simulink model "GS_model"  (R2018b)
settings: Solver=ode5  StartTime=0.0  StopTime=SimuStopTime  FixedStep=T_Simu  RelTol=1e-3
InitFcn:
  | Initial
undefined symbols (not defined in the file or in its folder): Aba10, Aba20, aeroCIP2006_S, aeroCIP2006_X, aeroCIP2006_Y, Agl0, Ass_kS, Ass_n1, Ass_n2, Ass_n3, Ass_n4, Ass_Noise, Ass_R, Ass_Resolution, Ass_TmOrder, AssA_Fix_Abs, AssB_Fix_Abs, AssC_Fix_Abs, AssD_Fix_Abs, AssE_Fix_Aps, AssF_Fix_Aps, C, c_max, c_min, Cd, CenterOfFigNX, CenterOfFigNY, CenterOfFigNZ, CenterOfFigP1, CenterOfFigP2, CenterOfFigPX, CenterOfFigPY, CenterOfFigPZ, Cmu, Crou, DEG2RAD, DiscIntNeverNeededParam, Eg_Dir, Eg_F, Eg_PrepareTime, Eg_r_L_L, Fw_Abf, Fw_Hmax, Fw_J, Fw_Spd0, Fw_Tmax, git_hash_BaseLine, git_hash_Project, Gnss_Noise_Pos, Gnss_Noise_Vel, Gnss_PropgationTime, GyroA_Fix_Abg, GyroA_Noise, GyroB_Fix_Abg, GyroB_Noise, GyroC_Fix_Abg, GyroC_Noise, GyroD_Fix_Abg, GyroD_Noise, h ... (+94)
libraries: simulink x308, sharedutil x46, aerolibutil x37, sharedtransform x31, vrlib x14, aerolibgravity2 x2
(part 2 of 20)

== system GS_model/Subsystem2/Tc/Fw2 ==
  FwSpd0 : Inport
  In1 : Inport  Port=2
  Constant : Constant  Value=[0;0;zeros(14,1);0]
  Constant1 : Constant  Value=TestMode
  Constant2 : Constant  Value=TestMode
  Constant3 : Constant  Value=Fw_Spd0
  Data Store Memory : DataStoreMemory  DataStoreName=Dyn_FWSpdSet  ReadBeforeWriteMsg=warning  WriteAfterWriteMsg=warning  WriteAfterReadMsg=warning  InitialValue=[0;0;0]  ShowAdditionalParam=off
  Data Store Memory1 : DataStoreMemory  DataStoreName=Dyn_FWCtrlSourceSet  ReadBeforeWriteMsg=warning  WriteAfterWriteMsg=warning  WriteAfterReadMsg=warning  InitialValue=[0;0]  ShowAdditionalParam=off
  Data Store Memory10 : DataStoreMemory  DataStoreName=Dyn_FWErr_TOP  ReadBeforeWriteMsg=warning  WriteAfterWriteMsg=warning  WriteAfterReadMsg=warning  InitialValue=[0;0]  ShowAdditionalParam=off
  Data Store Memory14 : DataStoreMemory  DataStoreName=Dyn_FwFricCoff  ReadBeforeWriteMsg=warning  WriteAfterWriteMsg=warning  WriteAfterReadMsg=warning  InitialValue=1  ShowAdditionalParam=off
  Data Store Memory17 : DataStoreMemory  DataStoreName=Dyn_FWTSet  ReadBeforeWriteMsg=warning  WriteAfterWriteMsg=warning  WriteAfterReadMsg=warning  InitialValue=[0;0;0]  ShowAdditionalParam=off
  Data Store Memory2 : DataStoreMemory  DataStoreName=Dyn_FWErr_SpdOP  ReadBeforeWriteMsg=warning  WriteAfterWriteMsg=warning  WriteAfterReadMsg=warning  InitialValue=[0;0]  ShowAdditionalParam=off
  Data Store Memory3 : DataStoreMemory  DataStoreName=FwSpd0  ReadBeforeWriteMsg=warning  WriteAfterWriteMsg=warning  WriteAfterReadMsg=warning  InitialValue=Fw_Spd0  ShowAdditionalParam=off
  Data Store Memory4 : DataStoreMemory  DataStoreName=Dyn_FwDelaySet  ReadBeforeWriteMsg=warning  WriteAfterWriteMsg=warning  WriteAfterReadMsg=warning  ShowAdditionalParam=off
  Data Store Memory6 : DataStoreMemory  DataStoreName=Dyn_FWModeSet  ReadBeforeWriteMsg=warning  WriteAfterWriteMsg=warning  WriteAfterReadMsg=warning  InitialValue=[0;0;0]  ShowAdditionalParam=off
  Data Store Read : DataStoreRead  DataStoreName=Dyn_FWSpdSet
  Data Store Read1 : DataStoreRead  DataStoreName=Dyn_FWCtrlSourceSet
  Data Store Read10 : DataStoreRead  DataStoreName=Dyn_FWErr_TOP
  Data Store Read14 : DataStoreRead  DataStoreName=Dyn_FwFricCoff
  Data Store Read17 : DataStoreRead  DataStoreName=Dyn_FWTSet
  Data Store Read2 : DataStoreRead  DataStoreName=Dyn_FWErr_SpdOP
  Data Store Read3 : DataStoreRead  DataStoreName=FwSpd0
  Data Store Read4 : DataStoreRead  DataStoreName=Dyn_FwDelaySet
  Data Store Read6 : DataStoreRead  DataStoreName=Dyn_FWModeSet
  Data Store Write : DataStoreWrite  DataStoreName=Dyn_FWSpdSet
  Data Store Write1 : DataStoreWrite  DataStoreName=Dyn_FWCtrlSourceSet
  Data Store Write10 : DataStoreWrite  DataStoreName=Dyn_FWErr_TOP
  Data Store Write14 : DataStoreWrite  DataStoreName=Dyn_FwFricCoff
  Data Store Write17 : DataStoreWrite  DataStoreName=Dyn_FWTSet
  Data Store Write2 : DataStoreWrite  DataStoreName=FwSpd0
  Data Store Write4 : DataStoreWrite  DataStoreName=Dyn_FwDelaySet
  Data Store Write6 : DataStoreWrite  DataStoreName=Dyn_FWModeSet
  Data Store Write8 : DataStoreWrite  DataStoreName=Dyn_FWErr_SpdOP
  Demux : Demux  Outputs=[2;1;3;3;3;2;2;1]
  Mux : Mux  Inputs=9
  Switch : Switch  Criteria=u2 > Threshold  Threshold=0.5
  Switch1 : Switch  Criteria=u2 > Threshold  Threshold=0.5
  Out1 : Outport
  wires:
  Mux/1 -> Out1/1
  Constant2/1 -> Switch/2
  Constant/1 -> Switch/1
  Switch/1 -> Demux/1
  Demux/1 -> Data Store Write1/1
  Demux/2 -> Data Store Write4/1
  Demux/3 -> Data Store Write17/1
  Demux/4 -> Data Store Write/1
  Demux/5 -> Data Store Write6/1
  Demux/6 -> Data Store Write8/1
  Demux/7 -> Data Store Write10/1
  Demux/8 -> Data Store Write14/1
  Data Store Read1/1 -> Mux/1
  Data Store Read4/1 -> Mux/2
  Data Store Read17/1 -> Mux/3
  Data Store Read/1 -> Mux/4
  Data Store Read6/1 -> Mux/5
  Data Store Read2/1 -> Mux/6
  Data Store Read10/1 -> Mux/7
  Data Store Read14/1 -> Mux/8
  Constant1/1 -> Switch1/2
  Switch1/1 -> Data Store Write2/1
  Constant3/1 -> Switch1/3
  FwSpd0/1 -> Switch1/1
  In1/1 -> Switch/3
  Data Store Read3/1 -> Mux/9

== system GS_model/Subsystem2/Tc/GNSS1 ==
  note: Dyn_GNSSGNDSet_Pos_Switch
      | Dyn_GNSSGNDSet_Pos_X
      | Dyn_GNSSGNDSet_Pos_Y
      | Dyn_GNSSGNDSet_Pos_Z
      | Dyn_GNSSErr_PosConstant_AxisChoice
      | Dyn_GNSSErr_PosConstant_Switch
      | Dyn_GNSSErr_PosWildValue_Switch
      | Dyn_GNSSGNDSet_Spd_Switch
      | Dyn_GNSSGNDSet_Spd_X
      | Dyn_GNSSGNDSet_Spd_Y
      | Dyn_GNSSGNDSet_Spd_Z
      | Dyn_GNSSErr_SpdConstant_AxisChoice
      | Dyn_GNSSErr_SpdConstant_Switch
      | Dyn_GNSSErr_SpdWildValue_Switch
      | Dyn_GNSS_T1
      | Dyn_GNSS_T2
  in : Inport
  Compare To Zero : simulink/Logic and Bit Operations/Compare To Zero  relop=~=  OutDataTypeStr=boolean
  Compare To Zero1 : simulink/Logic and Bit Operations/Compare To Zero  relop=~=  OutDataTypeStr=boolean
  Constant : Constant  Value=zeros(16,1)
  Constant2 : Constant  Value=TestMode
  Data Store Memory1 : DataStoreMemory  DataStoreName=Dyn_GNSSErr_SpdWildValue  ReadBeforeWriteMsg=warning  WriteAfterWriteMsg=warning  WriteAfterReadMsg=warning  ShowAdditionalParam=off
  Data Store Memory10 : DataStoreMemory  DataStoreName=Dyn_GNSSGNDSet_Spd  ReadBeforeWriteMsg=warning  WriteAfterWriteMsg=warning  WriteAfterReadMsg=warning  InitialValue=[0;0;0;0]  ShowAdditionalParam=off
  Data Store Memory14 : DataStoreMemory  DataStoreName=Dyn_GNSSErr_SpdConstant  ReadBeforeWriteMsg=warning  WriteAfterWriteMsg=warning  WriteAfterReadMsg=warning  InitialValue=[0;0]  ShowAdditionalParam=off
  Data Store Memory17 : DataStoreMemory  DataStoreName=Dyn_GNSSErr_PosConstant  ReadBeforeWriteMsg=warning  WriteAfterWriteMsg=warning  WriteAfterReadMsg=warning  InitialValue=[0;0]  ShowAdditionalParam=off
  Data Store Memory2 : DataStoreMemory  DataStoreName=Dyn_GNSS_PropagationTime1  ReadBeforeWriteMsg=warning  WriteAfterWriteMsg=warning  WriteAfterReadMsg=warning  InitialValue=Gnss_PropgationTime(1)  ShowAdditionalParam=off
  Data Store Memory3 : DataStoreMemory  DataStoreName=Dyn_GNSS_PropagationTime2  ReadBeforeWriteMsg=warning  WriteAfterWriteMsg=warning  WriteAfterReadMsg=warning  InitialValue=Gnss_PropgationTime(2)  ShowAdditionalParam=off
  Data Store Memory4 : DataStoreMemory  DataStoreName=Dyn_GNSSGNDSet_Pos  ReadBeforeWriteMsg=warning  WriteAfterWriteMsg=warning  WriteAfterReadMsg=warning  InitialValue=[0;0;0;0]  ShowAdditionalParam=off
  Data Store Memory8 : DataStoreMemory  DataStoreName=Dyn_GNSSErr_PosWildValue  ReadBeforeWriteMsg=warning  WriteAfterWriteMsg=warning  WriteAfterReadMsg=warning  ShowAdditionalParam=off
  Data Store Read1 : DataStoreRead  DataStoreName=Dyn_GNSSErr_SpdWildValue
  Data Store Read10 : DataStoreRead  DataStoreName=Dyn_GNSSGNDSet_Spd
  Data Store Read14 : DataStoreRead  DataStoreName=Dyn_GNSSErr_SpdConstant
  Data Store Read17 : DataStoreRead  DataStoreName=Dyn_GNSSErr_PosConstant
  Data Store Read2 : DataStoreRead  DataStoreName=Dyn_GNSS_PropagationTime1
  Data Store Read3 : DataStoreRead  DataStoreName=Dyn_GNSS_PropagationTime2
  Data Store Read4 : DataStoreRead  DataStoreName=Dyn_GNSSGNDSet_Pos
  Data Store Read8 : DataStoreRead  DataStoreName=Dyn_GNSSErr_PosWildValue
  Data Store Write1 : DataStoreWrite  DataStoreName=Dyn_GNSSErr_SpdWildValue
  Data Store Write10 : DataStoreWrite  DataStoreName=Dyn_GNSSGNDSet_Spd
  Data Store Write14 : DataStoreWrite  DataStoreName=Dyn_GNSSErr_SpdConstant
  Data Store Write17 : DataStoreWrite  DataStoreName=Dyn_GNSSErr_PosConstant
  Data Store Write4 : DataStoreWrite  DataStoreName=Dyn_GNSSGNDSet_Pos
  Data Store Write8 : DataStoreWrite  DataStoreName=Dyn_GNSSErr_PosWildValue
  Demux : Demux  Outputs=[4;2;1;4;2;1;1;1]
  Enabled Subsystem : Subsystem  TreatAsAtomicUnit=on
  Enabled Subsystem1 : Subsystem  TreatAsAtomicUnit=on
  Mux : Mux  Inputs=8
  Switch : Switch  Criteria=u2 > Threshold  Threshold=0.5
  Tc_GNSS : Outport
  wires:
  Switch/1 -> Demux/1
  Constant/1 -> Switch/1
  Constant2/1 -> Switch/2
  Mux/1 -> Tc_GNSS/1
  Demux/1 -> Data Store Write4/1
  Demux/2 -> Data Store Write17/1
  Demux/3 -> Data Store Write8/1
  Demux/4 -> Data Store Write10/1
  Demux/5 -> Data Store Write14/1
  Data Store Read8/1 -> Mux/3
  Data Store Read17/1 -> Mux/2
  Data Store Read10/1 -> Mux/4
  Data Store Read4/1 -> Mux/1
  Data Store Read14/1 -> Mux/5
  Demux/6 -> Data Store Write1/1
  Data Store Read1/1 -> Mux/6
  in/1 -> Switch/3
  Demux/7 -> Enabled Subsystem/1(In1), Compare To Zero/1
  Data Store Read2/1 -> Mux/7
  Compare To Zero/1 -> Enabled Subsystem/Enable
  Compare To Zero1/1 -> Enabled Subsystem1/Enable
  Demux/8 -> Compare To Zero1/1, Enabled Subsystem1/1(In1)
  Data Store Read3/1 -> Mux/8

== system GS_model/Subsystem2/Tc/Gyro1 ==
  note: Dyn_GyroGNDSet_Choice
      | Dyn_GyroGNDSet_Switch
      | Dyn_GyroGNDSet_wx
      | Dyn_GyroGNDSet_wy
      | Dyn_GyroGNDSet_wz
      | Dyn_GyroErr_Constant_Choice
      | Dyn_GyroErr_Constant_AxisChoice
      | Dyn_GyroErr_Constant_Switch
      | Dyn_GyroErr_WildValue_Choice
      | Dyn_GyroErr_WildValue_AxisChoice
      | Dyn_GyroErr_WildValue_Switch
      | Dyn_GyroErr_Jump_Choice
      | Dyn_GyroErr_Jump_AxisChoice
      | Dyn_GyroErr_Jump_Switch
      | Dyn_GyroErr_Jump_TSet
      | Dyn_GyroErr_Jump_AmpCoffSet
      | Dyn_GyroErr_Wave_Choice
      | Dyn_GyroErr_Wave_AxisChoice
      | Dyn_GyroErr_Wave_Switch
      | Dyn_GyroErr_Wave_AmpCoffSet
      | Dyn_GyroDriftSet_Choice
      | Dyn_GyroDriftSet_wx
      | Dyn_GyroDriftSet_wy
      | Dyn_GyroDriftSet_wz
  in : Inport
  Constant : Constant  Value=[zeros(15,1);1;0;0;0;0;zeros(4,1)]
  Constant2 : Constant  Value=TestMode
  Data Store Memory : DataStoreMemory  DataStoreName=Dyn_GyroGNDSet  ReadBeforeWriteMsg=warning  WriteAfterWriteMsg=warning  WriteAfterReadMsg=warning  InitialValue=[0;0;0;0;0]  ShowAdditionalParam=off
  Data Store Memory1 : DataStoreMemory  DataStoreName=Dyn_GyroDriftSet  ReadBeforeWriteMsg=warning  WriteAfterWriteMsg=warning  WriteAfterReadMsg=warning  InitialValue=[0;0;0;0]  ShowAdditionalParam=off
  Data Store Memory10 : DataStoreMemory  DataStoreName=Dyn_GyroErr_Jump  ReadBeforeWriteMsg=warning  WriteAfterWriteMsg=warning  WriteAfterReadMsg=warning  InitialValue=[0;0;0;0;1]  ShowAdditionalParam=off
  Data Store Memory14 : DataStoreMemory  DataStoreName=Dyn_GyroErr_Wave  ReadBeforeWriteMsg=warning  WriteAfterWriteMsg=warning  WriteAfterReadMsg=warning  InitialValue=[0;0;0;0]  ShowAdditionalParam=off
  Data Store Memory6 : DataStoreMemory  DataStoreName=Dyn_GyroErr_Constant  ReadBeforeWriteMsg=warning  WriteAfterWriteMsg=warning  WriteAfterReadMsg=warning  InitialValue=[0;0;0]  ShowAdditionalParam=off
  Data Store Memory8 : DataStoreMemory  DataStoreName=Dyn_GyroErr_WildValue  ReadBeforeWriteMsg=warning  WriteAfterWriteMsg=warning  WriteAfterReadMsg=warning  InitialValue=[0;0;0]  ShowAdditionalParam=off
  Data Store Read : DataStoreRead  DataStoreName=Dyn_GyroGNDSet
  Data Store Read1 : DataStoreRead  DataStoreName=Dyn_GyroDriftSet
  Data Store Read10 : DataStoreRead  DataStoreName=Dyn_GyroErr_Jump
  Data Store Read14 : DataStoreRead  DataStoreName=Dyn_GyroErr_Wave
  Data Store Read6 : DataStoreRead  DataStoreName=Dyn_GyroErr_Constant
  Data Store Read8 : DataStoreRead  DataStoreName=Dyn_GyroErr_WildValue
  Data Store Write : DataStoreWrite  DataStoreName=Dyn_GyroGNDSet
  Data Store Write1 : DataStoreWrite  DataStoreName=Dyn_GyroDriftSet
  Data Store Write10 : DataStoreWrite  DataStoreName=Dyn_GyroErr_Jump
  Data Store Write14 : DataStoreWrite  DataStoreName=Dyn_GyroErr_Wave
  Data Store Write6 : DataStoreWrite  DataStoreName=Dyn_GyroErr_Constant
  Data Store Write8 : DataStoreWrite  DataStoreName=Dyn_GyroErr_WildValue
  Demux : Demux  Outputs=[5;3;3;5;4;4]
  Mux : Mux  Inputs=6
  Switch : Switch  Criteria=u2 > Threshold  Threshold=0.5
  Tc_Gyro : Outport
  wires:
  Mux/1 -> Tc_Gyro/1
  Data Store Read8/1 -> Mux/3
  Demux/2 -> Data Store Write6/1
  Data Store Read10/1 -> Mux/4
  Data Store Read/1 -> Mux/1
  Data Store Read14/1 -> Mux/5
  Data Store Read6/1 -> Mux/2
  Demux/3 -> Data Store Write8/1
  Demux/4 -> Data Store Write10/1
  Demux/5 -> Data Store Write14/1
  Demux/1 -> Data Store Write/1
  Constant2/1 -> Switch/2
  Constant/1 -> Switch/1
  Switch/1 -> Demux/1
  Demux/6 -> Data Store Write1/1
  Data Store Read1/1 -> Mux/6
  in/1 -> Switch/3

== system GS_model/Subsystem2/Tc/High-Low-Bias1 ==
  in : Inport
  Constant : Constant  Value=[1;0;0;0]
  Constant2 : Constant  Value=TestMode
  Data Store Memory : DataStoreMemory  DataStoreName=Dyn_InertiaCoff  ReadBeforeWriteMsg=warning  WriteAfterWriteMsg=warning  WriteAfterReadMsg=warning  InitialValue=1  ShowAdditionalParam=off
  Data Store Memory6 : DataStoreMemory  DataStoreName=Dyn_CentDrift  ReadBeforeWriteMsg=warning  WriteAfterWriteMsg=warning  WriteAfterReadMsg=warning  InitialValue=[0;0;0]  ShowAdditionalParam=off
  Data Store Read : DataStoreRead  DataStoreName=Dyn_InertiaCoff
  Data Store Read6 : DataStoreRead  DataStoreName=Dyn_CentDrift
  Data Store Write : DataStoreWrite  DataStoreName=Dyn_InertiaCoff
  Data Store Write6 : DataStoreWrite  DataStoreName=Dyn_CentDrift
  Demux : Demux  Outputs=[1;3]
  Mux : Mux  Inputs=2
  Switch : Switch  Criteria=u2 > Threshold  Threshold=0.5
  Tc_Mt : Outport
  wires:
  in/1 -> Switch/3
  Mux/1 -> Tc_Mt/1
  Switch/1 -> Demux/1
  Data Store Read6/1 -> Mux/2
  Constant/1 -> Switch/1
  Data Store Read/1 -> Mux/1
  Demux/1 -> Data Store Write/1
  Constant2/1 -> Switch/2
  Demux/2 -> Data Store Write6/1

== system GS_model/Subsystem2/Tc/Mm1 ==
  note: Dyn_MmGNDSet_Choice
      | Dyn_MmGNDSet_Switch
      | Dyn_MmGNDSet_X
      | Dyn_MmGNDSet_Y
      | Dyn_MmGNDSet_Z
      | Dyn_MmErr_Constant_Choice
      | Dyn_MmErr_Constant_AxisChoice
      | Dyn_MmErr_Constant_Switch
      | Dyn_MmErr_Jump_Choice
      | Dyn_MmErr_Jump_AxisChoice
      | Dyn_MmErr_Jump_Switch
      | Dyn_MmErr_Jump_TSet
      | Dyn_MmErr_Jump_AmpCoffSet
      | Dyn_MmErr_Wave_Choice
      | Dyn_MmErr_Wave_AxisChoice
      | Dyn_MmErr_Wave_Switch
      | Dyn_MmErr_Wave_AmpCoffSet
      | Dyn_MmErr_WildValue_Choice
      | Dyn_MmErr_WildValue_AxisChoice
      | Dyn_MmErr_WildValue_Switch
  In1 : Inport
  Constant : Constant  Value=zeros(20,1)
  Constant2 : Constant  Value=TestMode
  Data Store Memory10 : DataStoreMemory  DataStoreName=Dyn_MmErr_Wave  ReadBeforeWriteMsg=warning  WriteAfterWriteMsg=warning  WriteAfterReadMsg=warning  InitialValue=[0;0;0;0]  ShowAdditionalParam=off
  Data Store Memory14 : DataStoreMemory  DataStoreName=Dyn_MmErr_WildValue  ReadBeforeWriteMsg=warning  WriteAfterWriteMsg=warning  WriteAfterReadMsg=warning  InitialValue=[0;0;0]  ShowAdditionalParam=off
  Data Store Memory17 : DataStoreMemory  DataStoreName=Dyn_MmErr_Constant  ReadBeforeWriteMsg=warning  WriteAfterWriteMsg=warning  WriteAfterReadMsg=warning  InitialValue=[0;0;0]  ShowAdditionalParam=off
  Data Store Memory4 : DataStoreMemory  DataStoreName=Dyn_MmGNDSet  ReadBeforeWriteMsg=warning  WriteAfterWriteMsg=warning  WriteAfterReadMsg=warning  InitialValue=[0;0;0;0;0]  ShowAdditionalParam=off
  Data Store Memory8 : DataStoreMemory  DataStoreName=Dyn_MmErr_Jump  ReadBeforeWriteMsg=warning  WriteAfterWriteMsg=warning  WriteAfterReadMsg=warning  InitialValue=zeros(5,1)  ShowAdditionalParam=off
  Data Store Read10 : DataStoreRead  DataStoreName=Dyn_MmErr_Wave
  Data Store Read14 : DataStoreRead  DataStoreName=Dyn_MmErr_WildValue
  Data Store Read17 : DataStoreRead  DataStoreName=Dyn_MmErr_Constant
  Data Store Read4 : DataStoreRead  DataStoreName=Dyn_MmGNDSet
  Data Store Read8 : DataStoreRead  DataStoreName=Dyn_MmErr_Jump
  Data Store Write10 : DataStoreWrite  DataStoreName=Dyn_MmErr_Wave
  Data Store Write14 : DataStoreWrite  DataStoreName=Dyn_MmErr_WildValue
  Data Store Write17 : DataStoreWrite  DataStoreName=Dyn_MmErr_Constant
  Data Store Write4 : DataStoreWrite  DataStoreName=Dyn_MmGNDSet
  Data Store Write8 : DataStoreWrite  DataStoreName=Dyn_MmErr_Jump
  Demux : Demux  Outputs=[5;3;5;4;3]
  Mux : Mux  Inputs=5
  Switch : Switch  Criteria=u2 > Threshold  Threshold=0.5
  Tc_Mm : Outport
  wires:
  Data Store Read14/1 -> Mux/5
  Data Store Read4/1 -> Mux/1
  Data Store Read10/1 -> Mux/4
  Data Store Read17/1 -> Mux/2
  Data Store Read8/1 -> Mux/3
  Demux/5 -> Data Store Write14/1
  Demux/4 -> Data Store Write10/1
  Demux/3 -> Data Store Write8/1
  Demux/2 -> Data Store Write17/1
  Demux/1 -> Data Store Write4/1
  Mux/1 -> Tc_Mm/1
  Constant2/1 -> Switch/2
  Constant/1 -> Switch/1
  Switch/1 -> Demux/1
  In1/1 -> Switch/3

== system GS_model/Subsystem2/Tc/Mt1 ==
  note: Dyn_MtCoffSet_1
      | Dyn_MtCoffSet_2
      | Dyn_MtCoffSet_3
      | Dyn_MtCoffSet_4
      | Dyn_MtCoffSet_5
      | Dyn_MtCoffSet_6
      | Dyn_MtGNDSet_Choice
      | Dyn_MtGNDSet_Switch
      | Dyn_MtGNDSet_Current
  in : Inport
  Constant : Constant  Value=[ones(6,1);0;0;0]
  Constant2 : Constant  Value=TestMode
  Data Store Memory : DataStoreMemory  DataStoreName=Dyn_MtCoffSet  ReadBeforeWriteMsg=warning  WriteAfterWriteMsg=warning  WriteAfterReadMsg=warning  InitialValue=[1;1;1;1;1;1]  ShowAdditionalParam=off
  Data Store Memory6 : DataStoreMemory  DataStoreName=Dyn_MtGNDSet  ReadBeforeWriteMsg=warning  WriteAfterWriteMsg=warning  WriteAfterReadMsg=warning  InitialValue=[0;0;0]  ShowAdditionalParam=off
  Data Store Read : DataStoreRead  DataStoreName=Dyn_MtCoffSet
  Data Store Read6 : DataStoreRead  DataStoreName=Dyn_MtGNDSet
  Data Store Write : DataStoreWrite  DataStoreName=Dyn_MtCoffSet
  Data Store Write6 : DataStoreWrite  DataStoreName=Dyn_MtGNDSet
  Demux : Demux  Outputs=[6;3]
  Mux : Mux  Inputs=2
  Switch : Switch  Criteria=u2 > Threshold  Threshold=0.5
  Tc_Mt : Outport
  wires:
  Demux/2 -> Data Store Write6/1
  Constant2/1 -> Switch/2
  Demux/1 -> Data Store Write/1
  Data Store Read/1 -> Mux/1
  Constant/1 -> Switch/1
  Data Store Read6/1 -> Mux/2
  Switch/1 -> Demux/1
  Mux/1 -> Tc_Mt/1
  in/1 -> Switch/3

== system GS_model/Subsystem2/Tc/Orbit ==
  note: a
      | e
      | i
      | OMG
      | ong
      | f
  In1 : Inport
  Clock : Clock
  Constant : Constant  Value=Orbit0
  Switch1 : Switch  Criteria=u2 > Threshold  Threshold=0.5
  Tc_Orbit0 : Outport
  wires:
  Constant/1 -> Switch1/3
  Clock/1 -> Switch1/2
  Switch1/1 -> Tc_Orbit0/1
  In1/1 -> Switch1/1

== system GS_model/Subsystem2/Tc/Orbit1 ==
  Orbit0 : Inport
  in : Inport  Port=2
  Constant12 : Constant  Value=TestMode
  Data Store Memory6 : DataStoreMemory  DataStoreName=Orbit0  ReadBeforeWriteMsg=warning  WriteAfterWriteMsg=warning  WriteAfterReadMsg=warning  InitialValue=Orbit0  ShowAdditionalParam=off
  Data Store Read6 : DataStoreRead  DataStoreName=Orbit0
  Data Store Write6 : DataStoreWrite  DataStoreName=Orbit0
  Switch : Switch  Criteria=u2 > Threshold  Threshold=0.5
  Tc_Orbit0 : Outport
  wires:
  Data Store Read6/1 -> Tc_Orbit0/1
  Constant12/1 -> Switch/2
  Switch/1 -> Data Store Write6/1
  Orbit0/1 -> Switch/1
  in/1 -> Switch/3

== system GS_model/Subsystem2/Tc/Panel ==
  note: Tc_PanelSpread
  note: PanelSpread0
  note: 3322
      | 遥控
  In1 : Inport
  Demux : Demux  Outputs=2
  Logical Operator : Logic  Operator=OR  AllPortsSameDT=off  OutDataTypeStr=boolean
  double→8lowbit : Subsystem
  double→8lowbit1 : Subsystem
  Tc_Spread0 : Outport
  wires:
  Demux/2 -> double→8lowbit1/1(In1)
  Logical Operator/1 -> Tc_Spread0/1
  Demux/1 -> double→8lowbit/1(In1)
  double→8lowbit1/1(Out1) -> Logical Operator/2
  double→8lowbit/1(Out1) -> Logical Operator/1
  In1/1 -> Demux/1

== system GS_model/Subsystem2/Tc/Panel2 ==
  note: 3322
      | 遥控
  Spread0 : Inport
  In : Inport  Port=2
  Constant1 : Constant  Value=TestMode
  Data Store Memory : DataStoreMemory  DataStoreName=Spread0  ReadBeforeWriteMsg=warning  WriteAfterWriteMsg=warning  WriteAfterReadMsg=warning  InitialValue=zeros(8,1)  ShowAdditionalParam=off
  Data Store Read : DataStoreRead  DataStoreName=Spread0
  Data Store Write : DataStoreWrite  DataStoreName=Spread0
  Switch : Switch  Criteria=u2 > Threshold  Threshold=0.5
  Tc_Spread0 : Outport
  wires:
  Switch/1 -> Data Store Write/1
  Constant1/1 -> Switch/2
  Spread0/1 -> Switch/1
  Data Store Read/1 -> Tc_Spread0/1
  In/1 -> Switch/3

== system GS_model/Subsystem2/Tc/QV ==
  note: AglQV0_1X
      | AglQV0_1Y
      | AglQV0_2X
      | AglQV0_2Y
      | Dyn_SpdCoffSet_QvA
      | Dyn_SpdCoffSet_QvB
      | Dyn_SpdCoffSet_QvC
      | Dyn_SpdCoffSet_QvD
      | Dyn_AglSet_Qv_Enable
      | Dyn_AglSet_QvA
      | Dyn_AglSet_QvB
      | Dyn_AglSet_QvC
      | Dyn_AglSet_QvD
      | QV_DataSource
  In1 : Inport
  Demux : Demux  Outputs=14
  Mux1 : Mux  Inputs=9
  Mux55 : Mux
  Tc_QV : Outport
  Tc_AglSet : Outport  Port=2
  Tc_DataSource : Outport  Port=3
  wires:
  Mux55/1 -> Tc_AglSet/1
  Mux1/1 -> Tc_QV/1
  In1/1 -> Demux/1
  Demux/1 -> Mux55/1
  Demux/2 -> Mux55/2
  Demux/3 -> Mux55/3
  Demux/4 -> Mux55/4
  Demux/5 -> Mux1/1
  Demux/6 -> Mux1/2
  Demux/7 -> Mux1/3
  Demux/8 -> Mux1/4
  Demux/9 -> Mux1/5
  Demux/10 -> Mux1/6
  Demux/11 -> Mux1/7
  Demux/12 -> Mux1/8
  Demux/13 -> Mux1/9
  Demux/14 -> Tc_DataSource/1

== system GS_model/Subsystem2/Tc/QV2 ==
  note: 按位取，从低到高为A~D
      | 1真0伪
  QV_Agl0 : Inport
  "Tc_QV " : Inport  Port=2
  Tc_AglSet : Inport  Port=3
  Tc_DataSource : Inport  Port=4
  Constant1 : Constant  Value=[0;0;0;0]
  Constant2 : Constant  Value=TestMode
  Constant3 : Constant  Value=[1;1;1;1;zeros(5,1)]
  Constant4 : Constant  Value=TestMode
  Constant5 : Constant  Value=TestMode
  Data Store Memory3 : DataStoreMemory  DataStoreName=AglQV0  ReadBeforeWriteMsg=warning  WriteAfterWriteMsg=warning  WriteAfterReadMsg=warning  InitialValue=[180;180;180;180]  ShowAdditionalParam=off
  Data Store Memory5 : DataStoreMemory  DataStoreName=QV_DataSource  ReadBeforeWriteMsg=warning  WriteAfterWriteMsg=warning  WriteAfterReadMsg=warning  InitialValue=[85;85;85;85]  ShowAdditionalParam=off
  Data Store Read1 : DataStoreRead  DataStoreName=QV_DataSource
  Data Store Read4 : DataStoreRead  DataStoreName=AglQV0
  Data Store Write : DataStoreWrite  DataStoreName=AglQV0
  Data Store Write1 : DataStoreWrite  DataStoreName=QV_DataSource
  Mux : Mux  Inputs=3
  Switch : Switch  Criteria=u2 > Threshold  Threshold=0.5
  Switch1 : Switch  Criteria=u2 > Threshold  Threshold=0.5
  Switch2 : Switch  Criteria=u2 > Threshold  Threshold=0.5
  double→4lowbit : Subsystem
  Tc_QV : Outport
  wires:
  Constant2/1 -> Switch/2
  QV_Agl0/1 -> Switch/1
  Tc_AglSet/1 -> Switch/3
  Constant4/1 -> Switch2/2
  "Tc_QV "/1 -> Switch2/3
  Constant3/1 -> Switch2/1
  Constant5/1 -> Switch1/2
  Switch1/1 -> Data Store Write1/1
  Constant1/1 -> Switch1/1
  double→4lowbit/1(Out1) -> Switch1/3
  Tc_DataSource/1 -> double→4lowbit/1(In1)
  Switch/1 -> Data Store Write/1
  Switch2/1 -> Mux/1
  Data Store Read4/1 -> Mux/2
  Mux/1 -> Tc_QV/1
  Data Store Read1/1 -> Mux/3

== system GS_model/Subsystem2/Tc/RemanMag1 ==
  In1 : Inport
  Constant : Constant  Value=RemanMag
  Constant1 : Constant  Value=TestMode
  Data Store Memory : DataStoreMemory  DataStoreName=RemanMag  ReadBeforeWriteMsg=warning  WriteAfterWriteMsg=warning  WriteAfterReadMsg=warning  InitialValue=[0;0;0]  ShowAdditionalParam=off
  Data Store Read : DataStoreRead  DataStoreName=RemanMag
  Data Store Write : DataStoreWrite  DataStoreName=RemanMag
  Switch : Switch  Criteria=u2 > Threshold  Threshold=0.5
  Tc_RemanMag : Outport
  wires:
  Data Store Read/1 -> Tc_RemanMag/1
  Constant1/1 -> Switch/2
  Switch/1 -> Data Store Write/1
  Constant/1 -> Switch/1
  In1/1 -> Switch/3

== system GS_model/Subsystem2/Tc/Reset1 ==
  Reset0 : Inport
  in : Inport  Port=2
  Constant1 : Constant  Value=TestMode
  Data Store Memory : DataStoreMemory  DataStoreName=Tc_Reset  ReadBeforeWriteMsg=warning  WriteAfterWriteMsg=warning  WriteAfterReadMsg=warning  InitialValue=hex2dec('33')  ShowAdditionalParam=off
  Data Store Read : DataStoreRead  DataStoreName=Tc_Reset
  Data Store Write : DataStoreWrite  DataStoreName=Tc_Reset
  Mux : Mux  Inputs=2
  Subsystem3 : Subsystem
  Switch : Switch  Criteria=u2 > Threshold  Threshold=0.5
  "Tc_Reset " : Outport
  wires:
  Reset0/1 -> Switch/1
  Subsystem3/1(OrbitReset) -> Mux/1
  Subsystem3/2(AttReset) -> Mux/2
  Constant1/1 -> Switch/2
  Mux/1 -> "Tc_Reset "/1
  Data Store Read/1 -> Subsystem3/1("command_word ")
  Switch/1 -> Data Store Write/1
  in/1 -> Switch/3

== system GS_model/Subsystem2/Tc/SADA ==
  note: AglSADA0_1A
      | AglSADA0_1B
      | AglSADA0_2A
      | AglSADA0_2B
      | AglSADA0_3A
      | AglSADA0_3B
      | Dyn_SpdCoffSet_SadaA
      | Dyn_SpdCoffSet_SadaB
      | Dyn_SpdCoffSet_SadaC
      | Dyn_SpdCoffSet_SadaD
      | Dyn_SpdCoffSet_SadaE
      | Dyn_SpdCoffSet_SadaF
      | Dyn_SADAErrSet_Choice
      | Dyn_SADAErrSet
      | Dyn_SADAErr_ReceiveCntConstant_Choice
      | Dyn_SADAErr_ReceiveCntConstant_Switch
      | Dyn_AglSet_Sada_Enable
      | Dyn_AglSet_SadaA
      | Dyn_AglSet_SadaB
      | Dyn_AglSet_SadaC
      | Dyn_AglSet_SadaD
      | Dyn_AglSet_SadaE
      | Dyn_AglSet_SadaF
      | Sada_DataSource
  In1 : Inport
  Demux : Demux  Outputs=24
  Mux1 : Mux  Inputs=6
  Mux11 : Mux  Inputs=12
  Mux55 : Mux  Inputs=6
  k1 : Gain  Gain=SADA_A_RotUnitSADA  SaturateOnIntegerOverflow=on  OutDataTypeStr=Inherit: Same as input  ParamDataTypeStr=Inherit: Same as input
  Tc_SADA : Outport
  Tc_AglSet : Outport  Port=2
  Tc_DataSource : Outport  Port=3
  wires:
  Mux11/1 -> Tc_SADA/1
  Mux55/1 -> Tc_AglSet/1
  Mux1/1 -> k1/1
  k1/1 -> Mux11/12
  In1/1 -> Demux/1
  Demux/1 -> Mux55/1
  Demux/2 -> Mux55/2
  Demux/3 -> Mux55/3
  Demux/4 -> Mux55/4
  Demux/5 -> Mux55/5
  Demux/6 -> Mux55/6
  Demux/7 -> Mux11/1
  Demux/8 -> Mux11/2
  Demux/9 -> Mux11/3
  Demux/10 -> Mux11/4
  Demux/11 -> Mux11/5
  Demux/12 -> Mux11/6
  Demux/13 -> Mux11/7
  Demux/14 -> Mux11/8
  Demux/15 -> Mux11/9
  Demux/16 -> Mux11/10
  Demux/17 -> Mux11/11
  Demux/18 -> Mux1/1
  Demux/19 -> Mux1/2
  Demux/20 -> Mux1/3
  Demux/21 -> Mux1/4
  Demux/22 -> Mux1/5
  Demux/23 -> Mux1/6
  Demux/24 -> Tc_DataSource/1

== system GS_model/Subsystem2/Tc/SADA2 ==
  note: 3322
  note: 按位取，从低到高为A~D
      | 1真0伪
  SADA_Agl0 : Inport
  "Tc_SADA " : Inport  Port=2
  Tc_AglSet : Inport  Port=3
  Tc_DataSource : Inport  Port=4
  Constant1 : Constant  Value=TestMode
  Constant2 : Constant  Value=TestMode
  Constant3 : Constant  Value=[1;1;1;1;1;1;zeros(11,1)]
  Constant4 : Constant  Value=TestMode
  Constant5 : Constant  Value=[0;0;0;0;0;0]
  Data Store Memory1 : DataStoreMemory  DataStoreName=AglSADA0  ReadBeforeWriteMsg=warning  WriteAfterWriteMsg=warning  WriteAfterReadMsg=warning  InitialValue=[-90;0;-90;0;0;0]  ShowAdditionalParam=off
  Data Store Memory2 : DataStoreMemory  DataStoreName=SADA_DataSource  ReadBeforeWriteMsg=warning  WriteAfterWriteMsg=warning  WriteAfterReadMsg=warning  InitialValue=[85;85;85;85;85;85]  ShowAdditionalParam=off
  Data Store Read1 : DataStoreRead  DataStoreName=SADA_DataSource
  Data Store Read4 : DataStoreRead  DataStoreName=AglSADA0
  Data Store Write : DataStoreWrite  DataStoreName=AglSADA0
  Data Store Write4 : DataStoreWrite  DataStoreName=SADA_DataSource
  Mux : Mux  Inputs=3
  Switch : Switch  Criteria=u2 > Threshold  Threshold=0.5
  Switch1 : Switch  Criteria=u2 > Threshold  Threshold=0.5
  Switch2 : Switch  Criteria=u2 > Threshold  Threshold=0.5
  double→4lowbit : Subsystem
  Tc_SADA : Outport
  wires:
  Constant2/1 -> Switch/2
  SADA_Agl0/1 -> Switch/1
  Tc_AglSet/1 -> Switch/3
  Constant4/1 -> Switch2/2
  "Tc_SADA "/1 -> Switch2/3
  Switch/1 -> Data Store Write/1
  Constant5/1 -> Switch1/1
  Constant1/1 -> Switch1/2
  Switch1/1 -> Data Store Write4/1
  double→4lowbit/1(Out1) -> Switch1/3
  Tc_DataSource/1 -> double→4lowbit/1(In1)
  Constant3/1 -> Switch2/1
  Switch2/1 -> Mux/1
  Data Store Read4/1 -> Mux/2
  Mux/1 -> Tc_SADA/1
  Data Store Read1/1 -> Mux/3

== system GS_model/Subsystem2/Tc/St1 ==
  note: Dyn_StValidSet_Choice
      | Dyn_StValidSet_Set
      | Dyn_StFixErr_Choice
      | Dyn_StFixErr_q0
      | Dyn_StFixErr_q1
      | Dyn_StFixErr_q2
      | Dyn_StFixErr_q3
      | Dyn_StNoiseCoff_Choice
      | Dyn_StNoiseCoff_Coff
      | Dyn_StGNDSet_Choice
      | Dyn_StGNDSet_Switch
      | Dyn_StGNDSet_q0
      | Dyn_StGNDSet_q1
      | Dyn_StGNDSet_q2
      | Dyn_StGNDSet_q3
      | Dyn_StErr_Constant_Choice
      | Dyn_StErr_Constant_Switch
      | Dyn_StErr_WildValue_Choice
      | Dyn_StErr_WildValue_Switch
      | Dyn_StErr_Jump_Choice
      | Dyn_StErr_Jump_Switch
      | Dyn_StErr_Jump_TSet
      | Dyn_StErr_Jump_AmpSet
      | Dyn_StErr_Wave_Choice
      | Dyn_StErr_Wave_Switch
      | Dyn_StErr_Wave_AmpCoffSet
  In1 : Inport
  Constant : Constant  Value=[[0;0];0;[1;0;0;0];0;1;0;0;[1;0;0;0];zeros(11,1)]
  Constant2 : Constant  Value=TestMode
  Data Store Memory : DataStoreMemory  DataStoreName=Dyn_StGNDSet  ReadBeforeWriteMsg=warning  WriteAfterWriteMsg=warning  WriteAfterReadMsg=warning  InitialValue=[0;0;1;0;0;0]  ShowAdditionalParam=off
  Data Store Memory1 : DataStoreMemory  DataStoreName=Dyn_StValidSet  ReadBeforeWriteMsg=warning  WriteAfterWriteMsg=warning  WriteAfterReadMsg=warning  InitialValue=[0;0]  ShowAdditionalParam=off
  Data Store Memory10 : DataStoreMemory  DataStoreName=Dyn_StErr_Jump  ReadBeforeWriteMsg=warning  WriteAfterWriteMsg=warning  WriteAfterReadMsg=warning  InitialValue=[0;0;0;0]  ShowAdditionalParam=off
  Data Store Memory14 : DataStoreMemory  DataStoreName=Dyn_StErr_Wave  ReadBeforeWriteMsg=warning  WriteAfterWriteMsg=warning  WriteAfterReadMsg=warning  InitialValue=[0;0;0]  ShowAdditionalParam=off
  Data Store Memory17 : DataStoreMemory  DataStoreName=Dyn_StNoiseCOF  ReadBeforeWriteMsg=warning  WriteAfterWriteMsg=warning  WriteAfterReadMsg=warning  InitialValue=[0;1]  ShowAdditionalParam=off
  Data Store Memory4 : DataStoreMemory  DataStoreName=Dyn_StFixErr  ReadBeforeWriteMsg=warning  WriteAfterWriteMsg=warning  WriteAfterReadMsg=warning  InitialValue=[0;1;0;0;0]  ShowAdditionalParam=off
  Data Store Memory6 : DataStoreMemory  DataStoreName=Dyn_StErr_Constant  ReadBeforeWriteMsg=warning  WriteAfterWriteMsg=warning  WriteAfterReadMsg=warning  InitialValue=[0;0]  ShowAdditionalParam=off
  Data Store Memory8 : DataStoreMemory  DataStoreName=Dyn_StErr_WildValue  ReadBeforeWriteMsg=warning  WriteAfterWriteMsg=warning  WriteAfterReadMsg=warning  InitialValue=[0;0]  ShowAdditionalParam=off
  Data Store Read : DataStoreRead  DataStoreName=Dyn_StGNDSet
  Data Store Read1 : DataStoreRead  DataStoreName=Dyn_StValidSet
  Data Store Read10 : DataStoreRead  DataStoreName=Dyn_StErr_Jump
  Data Store Read14 : DataStoreRead  DataStoreName=Dyn_StErr_Wave
  Data Store Read17 : DataStoreRead  DataStoreName=Dyn_StNoiseCOF
  Data Store Read4 : DataStoreRead  DataStoreName=Dyn_StFixErr
  Data Store Read6 : DataStoreRead  DataStoreName=Dyn_StErr_Constant
  Data Store Read8 : DataStoreRead  DataStoreName=Dyn_StErr_WildValue
  Data Store Write : DataStoreWrite  DataStoreName=Dyn_StGNDSet
  Data Store Write1 : DataStoreWrite  DataStoreName=Dyn_StValidSet
  Data Store Write10 : DataStoreWrite  DataStoreName=Dyn_StErr_Jump
  Data Store Write14 : DataStoreWrite  DataStoreName=Dyn_StErr_Wave
  Data Store Write17 : DataStoreWrite  DataStoreName=Dyn_StNoiseCOF
  Data Store Write4 : DataStoreWrite  DataStoreName=Dyn_StFixErr
  Data Store Write6 : DataStoreWrite  DataStoreName=Dyn_StErr_Constant
  Data Store Write8 : DataStoreWrite  DataStoreName=Dyn_StErr_WildValue
  Demux : Demux  Outputs=[2;5;2;6;2;2;4;3]
  Mux : Mux  Inputs=8
  Switch : Switch  Criteria=u2 > Threshold  Threshold=0.5
  Tc_St : Outport
  wires:
  Mux/1 -> Tc_St/1
  Demux/2 -> Data Store Write4/1
  Demux/3 -> Data Store Write17/1
  Demux/4 -> Data Store Write/1
  Demux/5 -> Data Store Write6/1
  Demux/6 -> Data Store Write8/1
  Demux/7 -> Data Store Write10/1
  Demux/8 -> Data Store Write14/1
  Data Store Read4/1 -> Mux/2
  Data Store Read17/1 -> Mux/3
  Data Store Read/1 -> Mux/4
  Data Store Read6/1 -> Mux/5
  Data Store Read8/1 -> Mux/6
  Data Store Read10/1 -> Mux/7
  Data Store Read14/1 -> Mux/8
  Constant2/1 -> Switch/2
  Constant/1 -> Switch/1
  Switch/1 -> Demux/1
  In1/1 -> Switch/3
  Demux/1 -> Data Store Write1/1
  Data Store Read1/1 -> Mux/1

== system GS_model/Subsystem2/Tc/TdCoffSet ==
  note: Dyn_AirDragCoffSet
      | Dyn_SunPressCoffSet
      | Dyn_DisTorque_CoffSet
  In1 : Inport
  Constant : Constant  Value=[1;1;1]
  Constant1 : Constant  Value=TestMode
  Data Store Memory : DataStoreMemory  DataStoreName=RemanMag  ReadBeforeWriteMsg=warning  WriteAfterWriteMsg=warning  WriteAfterReadMsg=warning  InitialValue=[0;0;0]  ShowAdditionalParam=off
  Data Store Read : DataStoreRead  DataStoreName=RemanMag
  Data Store Write : DataStoreWrite  DataStoreName=RemanMag
  Switch : Switch  Criteria=u2 > Threshold  Threshold=0.5
  Tc_TdCoffSet : Outport
  wires:
  Data Store Read/1 -> Tc_TdCoffSet/1
  Constant1/1 -> Switch/2
  Switch/1 -> Data Store Write/1
  Constant/1 -> Switch/1
  In1/1 -> Switch/3

== system GS_model/Subsystem2/Tc/TdCoffSet1 ==
  In1 : Inport
  Constant : Constant  Value=[1;1;1]
  Constant1 : Constant  Value=TestMode
  Data Store Memory : DataStoreMemory  DataStoreName=TdCoffSet  ReadBeforeWriteMsg=warning  WriteAfterWriteMsg=warning  WriteAfterReadMsg=warning  InitialValue=[0;0;0]  ShowAdditionalParam=off
  Data Store Read : DataStoreRead  DataStoreName=TdCoffSet
  Data Store Write : DataStoreWrite  DataStoreName=TdCoffSet
  Switch : Switch  Criteria=u2 > Threshold  Threshold=0.5
  Tc_TdCoffSet : Outport
  wires:
  Constant/1 -> Switch/1
  Switch/1 -> Data Store Write/1
  Constant1/1 -> Switch/2
  Data Store Read/1 -> Tc_TdCoffSet/1
  In1/1 -> Switch/3

== system GS_model/Subsystem2/Tc/Time1 ==
  YMDHMS : Inport
  in : Inport  Port=2
  Constant2 : Constant  Value=TestMode
  Data Store Memory : DataStoreMemory  DataStoreName=Tc_Time0  ReadBeforeWriteMsg=warning  WriteAfterWriteMsg=warning  WriteAfterReadMsg=warning  ShowAdditionalParam=off
  Data Store Read : DataStoreRead  DataStoreName=Tc_Time0
  Data Store Write : DataStoreWrite  DataStoreName=Tc_Time0
  Switch : Switch  Criteria=u2 > Threshold  Threshold=0.5
  YMDHMS 2 S : Subsystem
  Tc_Time0 : Outport
  wires:
  Data Store Read/1 -> Tc_Time0/1
  YMDHMS 2 S/1(UTC_1970) -> Switch/1
  Constant2/1 -> Switch/2
  Switch/1 -> Data Store Write/1
  YMDHMS/1 -> YMDHMS 2 S/1(YMDHMS)
  in/1 -> Switch/3

== system GS_model/Subsystem2/ /DynTelemetry/Subsystem ==
  Mux : Mux  Inputs=6
  Selector : Selector  NumberOfDimensions=2  InputPortWidth=9  IndexOptions=Index vector (dialog),Index vector (dialog)  Indices=1,1  OutputSizes=1,1
  Selector1 : Selector  NumberOfDimensions=2  InputPortWidth=9  IndexOptions=Index vector (dialog),Index vector (dialog)  Indices=2,2  OutputSizes=1,1
  Selector2 : Selector  NumberOfDimensions=2  InputPortWidth=9  IndexOptions=Index vector (dialog),Index vector (dialog)  Indices=3,3  OutputSizes=1,1
  Selector3 : Selector  NumberOfDimensions=2  InputPortWidth=9  IndexOptions=Index vector (dialog),Index vector (dialog)  Indices=1,2  OutputSizes=1,1
  Selector4 : Selector  NumberOfDimensions=2  InputPortWidth=9  IndexOptions=Index vector (dialog),Index vector (dialog)  Indices=1,3  OutputSizes=1,1
  Selector5 : Selector  NumberOfDimensions=2  InputPortWidth=9  IndexOptions=Index vector (dialog),Index vector (dialog)  Indices=2,3  OutputSizes=1,1
  Out1 : Outport  VectorParamsAs1DForOutWhenUnconnected=on
  wires:
  [I_sat] -> Selector5/1, Selector4/1, Selector3/1, Selector2/1, Selector1/1, Selector/1
  Selector/1 -> Mux/1
  Selector1/1 -> Mux/2
  Selector2/1 -> Mux/3
  Selector3/1 -> Mux/4
  Selector4/1 -> Mux/5
  Selector5/1 -> Mux/6
  Mux/1 -> Out1/1

== system GS_model/Subsystem2/ /DynTelemetry/TM_Orbit ==
  note: a
      | e
      | i
      | OMG
      | w
      | f
      | u
      | M
      | n
  Add : Sum
  Demux : Demux  Outputs=10
  Mux : Mux  Inputs=9
  Terminator : Terminator
  Terminator1 : Terminator
  Out1 : Outport  VectorParamsAs1DForOutWhenUnconnected=on
  wires:
  Demux/5 -> Add/1, Mux/5
  Demux/8 -> Terminator/1
  Demux/4 -> Mux/4
  Demux/7 -> Mux/8
  Add/1 -> Mux/7
  Demux/6 -> Mux/6, Add/2
  Demux/3 -> Mux/3
  Demux/2 -> Mux/2
  Demux/10 -> Mux/9
  Demux/9 -> Terminator1/1
  Demux/1 -> Mux/1
  [Orbit] -> Demux/1
  Mux/1 -> Out1/1

== system GS_model/Subsystem2/EquipmentCmd/Fw/Subsystem ==
  note: 422复杂动力学用，没mapping，暂时用udp替代
  note: 1 -- FW_Spd_422
      | 2 -- FW_Spd_UDP
      | 3 -- FW_Spd_FC
      |
      | 4 -- FW_T_422
      | 5 -- FW_T_UDP
      | 6 -- FW_T_FC
      |
      | 7 -- FW_Mode_422
      | 8 -- FW_Mode_UDP
      | 9 -- FW_Mode_FC
      |
      | 10--FW_DataSource
  In1 : Inport
  Demux : Demux  Outputs=7
  Mux2 : Mux  Inputs=10
  Cmd_FW : Outport
  wires:
  Demux/7 -> Mux2/10
  Demux/2 -> Mux2/3
  Demux/1 -> Mux2/2, Mux2/1
  Demux/6 -> Mux2/9
  Demux/5 -> Mux2/8, Mux2/7
  Demux/4 -> Mux2/6
  Demux/3 -> Mux2/5, Mux2/4
  Mux2/1 -> Cmd_FW/1
  In1/1 -> Demux/1

== system GS_model/Subsystem2/EquipmentCmd/Fw/Subsystem1 ==
  note: 1 -- FW_Spd_422
      | 2 -- FW_Spd_UDP
      | 3 -- FW_Spd_FC
      |
      | 4 -- FW_T_422
      | 5 -- FW_T_UDP
      | 6 -- FW_T_FC
      |
      | 7 -- FW_Mode_422
      | 8 -- FW_Mode_UDP
      | 9 -- FW_Mode_FC
      |
      | 10--FW_DataSource
  note: 422复杂动力学用，没mapping，暂时用udp替代
  In1 : Inport
  Demux : Demux  Outputs=7
  Mux2 : Mux  Inputs=10
  Cmd_FW : Outport
  wires:
  In1/1 -> Demux/1
  Mux2/1 -> Cmd_FW/1
  Demux/3 -> Mux2/4, Mux2/5
  Demux/4 -> Mux2/6
  Demux/5 -> Mux2/7, Mux2/8
  Demux/6 -> Mux2/9
  Demux/1 -> Mux2/1, Mux2/2
  Demux/2 -> Mux2/3
  Demux/7 -> Mux2/10

== system GS_model/Subsystem2/EquipmentCmd/Fw/Subsystem2 ==
  note: 422复杂动力学用，没mapping，暂时用udp替代
  note: 1 -- FW_Spd_422
      | 2 -- FW_Spd_UDP
      | 3 -- FW_Spd_FC
      |
      | 4 -- FW_T_422
      | 5 -- FW_T_UDP
      | 6 -- FW_T_FC
      |
      | 7 -- FW_Mode_422
      | 8 -- FW_Mode_UDP
      | 9 -- FW_Mode_FC
      |
      | 10--FW_DataSource
  In1 : Inport
  Demux : Demux  Outputs=7
  Mux2 : Mux  Inputs=10
  Cmd_FW : Outport
  wires:
  Demux/7 -> Mux2/10
  Demux/2 -> Mux2/3
  Demux/1 -> Mux2/2, Mux2/1
  Demux/6 -> Mux2/9
  Demux/5 -> Mux2/8, Mux2/7
  Demux/4 -> Mux2/6
  Demux/3 -> Mux2/5, Mux2/4
  Mux2/1 -> Cmd_FW/1
  In1/1 -> Demux/1

== system GS_model/Subsystem2/EquipmentCmd/Fw/Subsystem3 ==
  note: 1 -- FW_Spd_422
      | 2 -- FW_Spd_UDP
      | 3 -- FW_Spd_FC
      |
      | 4 -- FW_T_422
      | 5 -- FW_T_UDP
      | 6 -- FW_T_FC
      |
      | 7 -- FW_Mode_422
      | 8 -- FW_Mode_UDP
      | 9 -- FW_Mode_FC
      |
      | 10--FW_DataSource
  note: 422复杂动力学用，没mapping，暂时用udp替代
  In1 : Inport
  Demux : Demux  Outputs=7
  Mux2 : Mux  Inputs=10
  Cmd_FW : Outport
  wires:
  In1/1 -> Demux/1
  Mux2/1 -> Cmd_FW/1
  Demux/3 -> Mux2/4, Mux2/5
  Demux/4 -> Mux2/6
  Demux/5 -> Mux2/7, Mux2/8
  Demux/6 -> Mux2/9
  Demux/1 -> Mux2/1, Mux2/2
  Demux/2 -> Mux2/3
  Demux/7 -> Mux2/10

== system GS_model/Subsystem2/EquipmentCmd/Fw/Subsystem4 ==
  note: 422复杂动力学用，没mapping，暂时用udp替代
  note: 1 -- FW_Spd_422
      | 2 -- FW_Spd_UDP
      | 3 -- FW_Spd_FC
      |
      | 4 -- FW_T_422
      | 5 -- FW_T_UDP
      | 6 -- FW_T_FC
      |
      | 7 -- FW_Mode_422
      | 8 -- FW_Mode_UDP
      | 9 -- FW_Mode_FC
      |
      | 10--FW_DataSource
  In1 : Inport
  Demux : Demux  Outputs=7
  Mux2 : Mux  Inputs=10
  Cmd_FW : Outport
  wires:
  Demux/7 -> Mux2/10
  Demux/2 -> Mux2/3
  Demux/1 -> Mux2/2, Mux2/1
  Demux/6 -> Mux2/9
  Demux/5 -> Mux2/8, Mux2/7
  Demux/4 -> Mux2/6
  Demux/3 -> Mux2/5, Mux2/4
  Mux2/1 -> Cmd_FW/1
  In1/1 -> Demux/1

== system GS_model/Subsystem2/EquipmentCmd/Fw/Subsystem5 ==
  note: 1 -- FW_Spd_422
      | 2 -- FW_Spd_UDP
      | 3 -- FW_Spd_FC
      |
      | 4 -- FW_T_422
      | 5 -- FW_T_UDP
      | 6 -- FW_T_FC
      |
      | 7 -- FW_Mode_422
      | 8 -- FW_Mode_UDP
      | 9 -- FW_Mode_FC
      |
      | 10--FW_DataSource
  note: 422复杂动力学用，没mapping，暂时用udp替代
  In1 : Inport
  Demux : Demux  Outputs=7
  Mux2 : Mux  Inputs=10
  Cmd_FW : Outport
  wires:
  In1/1 -> Demux/1
  Mux2/1 -> Cmd_FW/1
  Demux/3 -> Mux2/4, Mux2/5
  Demux/4 -> Mux2/6
  Demux/5 -> Mux2/7, Mux2/8
  Demux/6 -> Mux2/9
  Demux/1 -> Mux2/1, Mux2/2
  Demux/2 -> Mux2/3
  Demux/7 -> Mux2/10

== system GS_model/Subsystem2/EquipmentCmd/Fw1/Subsystem7 ==
  note: FW_DataSource
      | AA-真采集（默认）  1-422(DB9);
      |                                  0-反测（默认
      | 55 -伪采集                UDP
  Tc_Fw : Inport
  FwA_Cmd : Inport  Port=2
  FwB_Cmd : Inport  Port=3
  FwC_Cmd : Inport  Port=4
  FwD_Cmd : Inport  Port=5
  FwE_Cmd : Inport  Port=6
  FwF_Cmd : Inport  Port=7
  Constant : Constant
  Constant1 : Constant  Value=2
  Constant2 : Constant  Value=3
  Constant3 : Constant  Value=4
  Constant4 : Constant  Value=5
  Constant5 : Constant  Value=6
  Mux : Mux  Inputs=6
  Subsystem1 : Subsystem
  Subsystem2 : Subsystem
  Subsystem3 : Subsystem
  Subsystem4 : Subsystem
  Subsystem5 : Subsystem
  Subsystem6 : Subsystem
  Fw_Mode/Spd/T : Outport
  wires:
  FwA_Cmd/1 -> Subsystem6/2(FW_Cmd)
  Constant/1 -> Subsystem6/1(FWNum)
  Tc_Fw/1 -> Subsystem1/3(TC_Fw), Subsystem2/3(TC_Fw), Subsystem3/3(TC_Fw), Subsystem5/3(TC_Fw), Subsystem4/3(TC_Fw), Subsystem6/3(TC_Fw)
  FwB_Cmd/1 -> Subsystem1/2(FW_Cmd)
  FwC_Cmd/1 -> Subsystem2/2(FW_Cmd)
  FwD_Cmd/1 -> Subsystem3/2(FW_Cmd)
  FwE_Cmd/1 -> Subsystem4/2(FW_Cmd)
  FwF_Cmd/1 -> Subsystem5/2(FW_Cmd)
  Constant1/1 -> Subsystem1/1(FWNum)
  Constant2/1 -> Subsystem2/1(FWNum)
  Constant3/1 -> Subsystem3/1(FWNum)
  Constant4/1 -> Subsystem4/1(FWNum)
  Constant5/1 -> Subsystem5/1(FWNum)
  Subsystem1/1(Cmd_Mode/Spd/T) -> Mux/2
  Subsystem6/1(Cmd_Mode/Spd/T) -> Mux/1
  Subsystem2/1(Cmd_Mode/Spd/T) -> Mux/3
  Subsystem3/1(Cmd_Mode/Spd/T) -> Mux/4
  Subsystem4/1(Cmd_Mode/Spd/T) -> Mux/5
  Subsystem5/1(Cmd_Mode/Spd/T) -> Mux/6
  Mux/1 -> Fw_Mode/Spd/T/1

== system GS_model/Subsystem2/EquipmentCmd/Mt1/Cmd_Mt_Analysis ==
  note: 55--UDP
      | AA--FC
  udp_Mt : Inport
  FC_Mt : Inport  Port=2
  Mt_Data_Source : Inport  Port=3
  Add1 : Sum
  Constant : Constant  Value=85
  Constant1 : Constant  Value=170
  Data Type Conversion1 : DataTypeConversion  OutDataTypeStr=double  SaturateOnIntegerOverflow=on  RndMeth=Zero
  Data Type Conversion3 : DataTypeConversion  OutDataTypeStr=double  SaturateOnIntegerOverflow=on  RndMeth=Zero
  Product1 : Product  SaturateOnIntegerOverflow=on  OutDataTypeStr=Inherit: Same as first input
  Product11 : Product  SaturateOnIntegerOverflow=on  OutDataTypeStr=Inherit: Same as first input
  Relational Operator : RelationalOperator  Operator===  RndMeth=Nearest
  Relational Operator2 : RelationalOperator  Operator===  RndMeth=Nearest
  Cmd_Mt_Pro : Outport
  wires:
  udp_Mt/1 -> Product1/1
  Data Type Conversion3/1 -> Product11/2
  Constant/1 -> Relational Operator/2
  Add1/1 -> Cmd_Mt_Pro/1
  FC_Mt/1 -> Product11/1
  Data Type Conversion1/1 -> Product1/2
  Constant1/1 -> Relational Operator2/2
  Mt_Data_Source/1 -> Relational Operator/1, Relational Operator2/1
  Product11/1 -> Add1/1
  Relational Operator/1 -> Data Type Conversion1/1
  Product1/1 -> Add1/2
  Relational Operator2/1 -> Data Type Conversion3/1

== system GS_model/Subsystem2/EquipmentCmd/PanelSpread/double→8lowbit ==
  In1 : Inport
  Bitwise Operator : simulink/Logic and Bit Operations/Bitwise Operator  logicop=AND  UseBitMask=on  BitMask=bin2dec('00000001')  BitMaskRealWorld=Stored Integer
  Bitwise Operator1 : simulink/Logic and Bit Operations/Bitwise Operator  logicop=AND  UseBitMask=on  BitMask=bin2dec('00000010')  BitMaskRealWorld=Stored Integer
  Bitwise Operator2 : simulink/Logic and Bit Operations/Bitwise Operator  logicop=AND  UseBitMask=on  BitMask=bin2dec('00000100')  BitMaskRealWorld=Stored Integer
  Bitwise Operator3 : simulink/Logic and Bit Operations/Bitwise Operator  logicop=AND  UseBitMask=on  BitMask=bin2dec('00001000')  BitMaskRealWorld=Stored Integer
  Bitwise Operator4 : simulink/Logic and Bit Operations/Bitwise Operator  logicop=AND  UseBitMask=on  BitMask=bin2dec('00010000')  BitMaskRealWorld=Stored Integer
  Bitwise Operator5 : simulink/Logic and Bit Operations/Bitwise Operator  logicop=AND  UseBitMask=on  BitMask=bin2dec('00100000')  BitMaskRealWorld=Stored Integer
  Bitwise Operator6 : simulink/Logic and Bit Operations/Bitwise Operator  logicop=AND  UseBitMask=on  BitMask=bin2dec('01000000')  BitMaskRealWorld=Stored Integer
  Bitwise Operator7 : simulink/Logic and Bit Operations/Bitwise Operator  logicop=AND  UseBitMask=on  BitMask=bin2dec('10000000')  BitMaskRealWorld=Stored Integer
  Compare To Zero{,1..7} (8 alike) : simulink/Logic and Bit Operations/Compare To Zero  relop=>  OutDataTypeStr=boolean
  Data Type Conversion : DataTypeConversion  OutDataTypeStr=uint8
  Mux : Mux  Inputs=8
  Out1 : Outport
  wires:
  Data Type Conversion/1 -> Bitwise Operator7/1, Bitwise Operator6/1, Bitwise Operator5/1, Bitwise Operator4/1, Bitwise Operator3/1, Bitwise Operator2/1, Bitwise Operator1/1, Bitwise Operator/1
  Bitwise Operator1/1 -> Compare To Zero1/1
  Compare To Zero1/1 -> Mux/2
  Compare To Zero/1 -> Mux/1
  Bitwise Operator/1 -> Compare To Zero/1
  In1/1 -> Data Type Conversion/1
  Mux/1 -> Out1/1
  Bitwise Operator2/1 -> Compare To Zero2/1
  Bitwise Operator3/1 -> Compare To Zero3/1
  Bitwise Operator4/1 -> Compare To Zero4/1
  Bitwise Operator5/1 -> Compare To Zero5/1
  Bitwise Operator6/1 -> Compare To Zero6/1
  Bitwise Operator7/1 -> Compare To Zero7/1
  Compare To Zero2/1 -> Mux/3
  Compare To Zero3/1 -> Mux/4
  Compare To Zero4/1 -> Mux/5
  Compare To Zero5/1 -> Mux/6
  Compare To Zero6/1 -> Mux/7
  Compare To Zero7/1 -> Mux/8

== system GS_model/Subsystem2/Subsystem/Actuator/Engine ==
  Tc_F_Engine : Inport
  Cmd_Engine : Inport  Port=2
  Cent : Inport  Port=3
  Constant : Constant  Value=Eg_r_L_L  VectorParams1D=off
  Constant1 : Constant  Value=Eg_F
  Constant2 : Constant
  Constant3 : Constant  Value=Eg_PrepareTime
  Constant4 : Constant  Value=Eg_Dir
  Constant5 : Constant  Value=2
  Subsystem : Subsystem
  Subsystem1 : Subsystem
  Sum : Sum
  Sum1 : Sum
  T_Engine : Outport
  F_EP : Outport  Port=2
  wires:
  Tc_F_Engine/1 -> Subsystem1/1(Tc_F_Engine), Subsystem/1(Tc_F_Engine)
  Cent/1 -> Subsystem1/3(Cent), Subsystem/3(Cent)
  Constant2/1 -> Subsystem/8(EgNum)
  Constant1/1 -> Subsystem1/4(Eg_F), Subsystem/4(Eg_F)
  Constant/1 -> Subsystem1/6(Eg_r_L_L), Subsystem/6(Eg_r_L_L)
  Cmd_Engine/1 -> Subsystem1/2(Cmd_Engine), Subsystem/2(Cmd_Engine)
  Constant3/1 -> Subsystem1/5(Eg_PrepareTime), Subsystem/5(Eg_PrepareTime)
  Constant4/1 -> Subsystem1/7(Eg_Dir), Subsystem/7(Eg_Dir)
  Constant5/1 -> Subsystem1/8(EgNum)
  Subsystem/1(T) -> Sum/1
  Subsystem1/1(T) -> Sum/2
  Subsystem/2(F) -> Sum1/1
  Subsystem1/2(F) -> Sum1/2
  Sum/1 -> T_Engine/1
  Sum1/1 -> F_EP/1
